simulink library "SimulinkLibrary"  (R2021b)
settings: Solver=VariableStepAuto  StartTime=0.0  StopTime=10.0  RelTol=1e-3
undefined symbols (not defined in the file): Ts, w0
libraries: canmsglib x6, $bdroot x5, sharedtransform x2, simulink x1
(part 2 of 3)

== system SimulinkLibrary/Sec ==
  SecContns : Inport
  Constant : Constant  Value=59  OutDataTypeStr=Inherit: Inherit via back propagation
  Constant1 : Constant  Value=0  OutDataTypeStr=Inherit: Inherit via back propagation
  Constant2 : Constant  Value=59  OutDataTypeStr=Inherit: Inherit via back propagation
  CountTo60 : Stateflow chart  TreatAsAtomicUnit=on
  Data Type Conversion1 : DataTypeConversion  OutDataTypeStr=boolean
  Equal : RelationalOperator  Operator===  OutDataTypeStr=boolean  RndMeth=Simplest
  Floor : Rounding
  Logical Operator : Logic  AllPortsSameDT=off  OutDataTypeStr=boolean
  Min : MinMax  Inputs=2
  Subtract : Sum  Inputs=+-
  Switch : Switch  Criteria=u2 ~= 0
  Unit Delay : UnitDelay  SampleTime=-1  HasFrameUpgradeWarning=on
  Unit Delay1 : UnitDelay  SampleTime=-1  HasFrameUpgradeWarning=on
  Sec : Outport
  wires:
  Constant1/1 -> Switch/1
  Constant/1 -> Min/2
  Floor/1 -> Unit Delay/1, Subtract/1  "floor"
  Logical Operator/1 -> Switch/2
  CountTo60/1(Out) -> Min/1  "Out"
  Min/1 -> Unit Delay1/1, Switch/3
  Constant2/1 -> Equal/2
  Unit Delay1/1 -> Equal/1
  Subtract/1 -> CountTo60/1(In), Data Type Conversion1/1  "In"
  Switch/1 -> Sec/1  "Seconds"
  Equal/1 -> Logical Operator/1
  SecContns/1 -> Floor/1  "SecContns"
  Unit Delay/1 -> Subtract/2
  Data Type Conversion1/1 -> Logical Operator/2

== system SimulinkLibrary/Vehicle Longitudinal model 1DOF ==
  FwF : Inport
  FwR : Inport  Port=2
  Grade : Inport  Port=3
  WindX : Inport  Port=4
  AirTempConstant : Constant  Value=T
  FExtConstant : Constant  Value=[0,0,0]
  MExtConstant : Constant  Value=[0,0,0]
  Subsystem : Subsystem
  Info : Outport  VectorParamsAs1DForOutWhenUnconnected=off
  xdot : Outport  Port=2  PortDimensions=1  VectorParamsAs1DForOutWhenUnconnected=off
  FzF : Outport  Port=3  PortDimensions=1  VectorParamsAs1DForOutWhenUnconnected=off
  FzR : Outport  Port=4  PortDimensions=1  VectorParamsAs1DForOutWhenUnconnected=off
  wires:
  Subsystem/4(FzR) -> FzR/1
  FwF/1 -> Subsystem/1(FwF)
  FwR/1 -> Subsystem/2(FwR)
  Subsystem/1(Info) -> Info/1
  AirTempConstant/1 -> Subsystem/7(Temp)
  WindX/1 -> Subsystem/4(wind)
  MExtConstant/1 -> Subsystem/6(MExt)
  Subsystem/3(FzF) -> FzF/1
  FExtConstant/1 -> Subsystem/5(FExt)
  Grade/1 -> Subsystem/3(Grade)
  Subsystem/2(xdot) -> xdot/1

== system SimulinkLibrary/Bundles/HwSelProc ==
  EX_DrvBtn_B_Psd : Inport
  EX_RvrsBtn_B_Psd : Inport  Port=2
  EX_NeutBtn_B_Psd : Inport  Port=3
  GearSelHeal_T_Pt : Inport  Port=4
  GearSelTrig_T_Pt : Inport  Port=5
  DMS_GearLock_B_Reqd : Inport  Port=6
  Chart : Stateflow chart  TreatAsAtomicUnit=on
  Chart1 : Stateflow chart  TreatAsAtomicUnit=on
  Chart2 : Stateflow chart  TreatAsAtomicUnit=on
  Chart3 : Stateflow chart  TreatAsAtomicUnit=on
      settings: PortSchema="{\"entries\":[{\"content\":{\"sides\":[{\"content\":{\"connectorIds\":[\"In2\",\"In1\",\"In3\",\"In4\"]},\"type\":\"ConnectorPlacement.EquallySpacedRectSide\",\"uuid\":\"b0ed4c9f-00b8-42d9-8b9d-c324759176df\"},{\"content\":{\"connectorIds\":[\"Out1\"],\"side\":\"RIGHT\"},\"type\":\"ConnectorPlacement.EquallySpacedRectSide\",\"uuid\":\"c1b9fe74-1ccd-4df0-a60b-616e1fa68e70\"},{\"content\":{\"connectorIds\":[],\"side\":\"TOP\"},\"type\":\"ConnectorPlacement.EquallySpacedRectSide\",\"uuid\":\"07870c33-9b1f-4d61-9115-d019d8c5b702\"}]},\"type\":\"ConnectorPlacement.EquallySpacedConnector\",\"uuid\":\"fdc9da14-557c-4fc0-875a-2215d5d98432\"}],\"packageUris\":[\"http://schema.mathworks.com/mf0/Connector/R2020b\"],\"version\":\"1.0\"}"
  DMS_HwEltGearPosn_Zs : Outport
  wires:
  Chart3/1(DMS_HwEltGearPosn_Zs) -> DMS_HwEltGearPosn_Zs/1
  DMS_GearLock_B_Reqd/1 -> Chart3/4(DMS_GearLock_B_Reqd)  "DMS_GearLock_B_Reqd"
  Chart2/1(Out) -> Chart3/3(NeutBtn_B_PsdFild)  "NeutBtn_B_PsdFild"
  Chart1/1(Out) -> Chart3/1(DrvBtn_B_PsdFild)  "DrvBtn_B_PsdFild"
  Chart/1(Out) -> Chart3/2(RvrsBtn_B_PsdFild)  "DrvBtn_B_PsdFild"
  [GearSelTrig_T_Pt] -> Chart2/3(TriggerTime)
  [GearSelHeal_T_Pt] -> Chart2/2(HealTime)
  [GearSelTrig_T_Pt] -> Chart1/3(TriggerTime)
  [GearSelHeal_T_Pt] -> Chart1/2(HealTime)
  [GearSelTrig_T_Pt] -> Chart/3(TriggerTime)
  [GearSelHeal_T_Pt] -> Chart/2(HealTime)
  EX_NeutBtn_B_Psd/1 -> Chart2/1(In)  "EX_NeutBtn_B_Psd"
  EX_RvrsBtn_B_Psd/1 -> Chart1/1(In)  "EX_RvrsBtn_B_Psd"
  EX_DrvBtn_B_Psd/1 -> Chart/1(In)  "EX_DrvBtn_B_Psd"
  GearSelHeal_T_Pt/1 -> [GearSelHeal_T_Pt]  "GearSelHeal_T_Pt"
  GearSelTrig_T_Pt/1 -> [GearSelTrig_T_Pt]  "GearSelTrig_T_Pt"

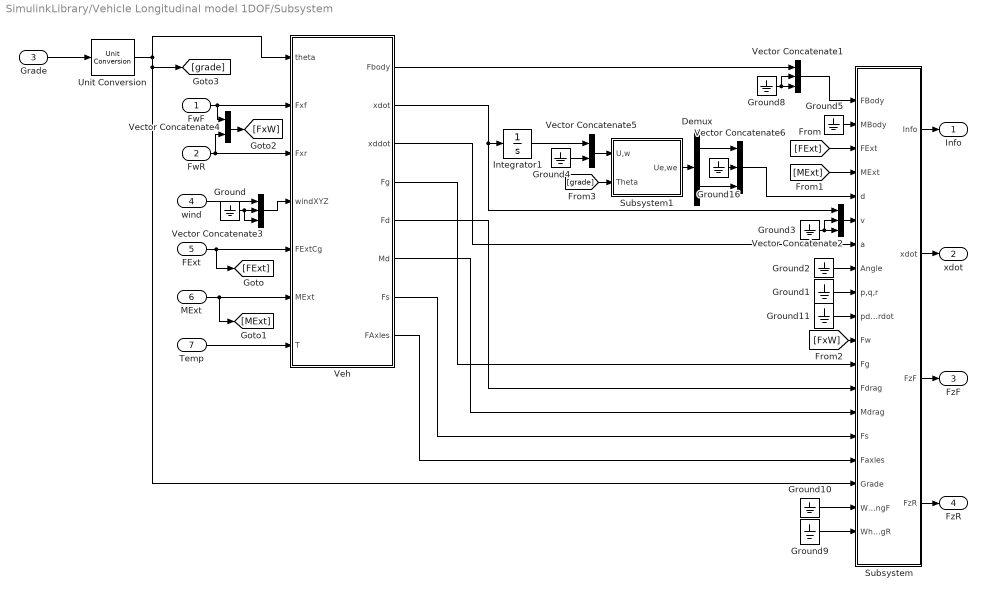
== system SimulinkLibrary/Vehicle Longitudinal model 1DOF/Subsystem ==
  FwF : Inport  Unit=N
  FwR : Inport  Port=2  Unit=N
  Grade : Inport  Port=3  Unit=deg
  wind : Inport  Port=4  Unit=m/s
  FExt : Inport  Port=5  Unit=N
  MExt : Inport  Port=6  Unit=N*m
  Temp : Inport  Port=7  OutMin=eps  Unit=K
  Demux : Demux  Outputs=2
  Ground{,1..5,8..11,16} (11 alike) : Ground
  Integrator1 : Integrator  InitialCondition=x_o
  Subsystem : Subsystem
  Subsystem1 : Subsystem
  Unit Conversion : UnitConversion
  Vector Concatenate{1..3,6} (4 alike) : Concatenate  NumInputs=3
  Vector Concatenate4 : Concatenate
  Vector Concatenate5 : Concatenate
  Veh : Subsystem
  Info : Outport  VectorParamsAs1DForOutWhenUnconnected=off
  xdot : Outport  Port=2  Unit=m/s  VectorParamsAs1DForOutWhenUnconnected=off
  FzF : Outport  Port=3  Unit=N  VectorParamsAs1DForOutWhenUnconnected=off
  FzR : Outport  Port=4  Unit=N  VectorParamsAs1DForOutWhenUnconnected=off
  wires:
  MExt/1 -> Veh/6(MExt), [MExt]
  [MExt] -> Subsystem/4(MExt)
  Veh/7(Fs) -> Subsystem/15(Fs)
  Ground9/1 -> Subsystem/19(WhlAngR)
  Vector Concatenate5/1 -> Subsystem1/1(U,w)
  Ground4/1 -> Vector Concatenate5/2
  Ground16/1 -> Vector Concatenate6/2
  Veh/4(Fg) -> Subsystem/12(Fg)
  Demux/1 -> Vector Concatenate6/1
  Subsystem1/1(Ue,we) -> Demux/1
  Vector Concatenate3/1 -> Veh/4(windXYZ)
  Veh/5(Fd) -> Subsystem/13(Fdrag)
  Unit Conversion/1 -> Veh/1(theta), Subsystem/17(Grade), [grade]
  Ground5/1 -> Subsystem/2(MBody)
  [FxW] -> Subsystem/11(Fw)
  Ground11/1 -> Subsystem/10(pdot,qdot,rdot)
  Vector Concatenate2/1 -> Subsystem/6(v)
  Veh/3(xddot) -> Subsystem/7(a)
  Veh/6(Md) -> Subsystem/14(Mdrag)
  Demux/2 -> Vector Concatenate6/3
  FwF/1 -> Veh/2(Fxf), Vector Concatenate4/1
  Ground1/1 -> Subsystem/9(p,q,r)
  Subsystem/1(Info) -> Info/1
  Ground10/1 -> Subsystem/18(WhlAngF)
  FwR/1 -> Veh/3(Fxr), Vector Concatenate4/2
  Subsystem/4(FzR) -> FzR/1
  Vector Concatenate4/1 -> [FxW]
  Veh/8(FAxles) -> Subsystem/16(Faxles)
  Veh/2(xdot) -> Integrator1/1, Vector Concatenate2/1
  Ground3/1 -> Vector Concatenate2/3, Vector Concatenate2/2
  Grade/1 -> Unit Conversion/1
  Subsystem/2(xdot) -> xdot/1
  Subsystem/3(FzF) -> FzF/1
  Ground2/1 -> Subsystem/8(Angle)
  Integrator1/1 -> Vector Concatenate5/1
  [FExt] -> Subsystem/3(FExt)
  Vector Concatenate1/1 -> Subsystem/1(FBody)
  FExt/1 -> Veh/5(FExtCg), [FExt]
  Veh/1(Fbody) -> Vector Concatenate1/1
  Temp/1 -> Veh/7(T)
  Vector Concatenate6/1 -> Subsystem/5(d)
  [grade] -> Subsystem1/2(Theta)
  Ground8/1 -> Vector Concatenate1/2, Vector Concatenate1/3
  wind/1 -> Vector Concatenate3/1
  Ground/1 -> Vector Concatenate3/3, Vector Concatenate3/2

== system SimulinkLibrary/Vehicle Longitudinal model 1DOF/Subsystem/Subsystem ==
  FBody : Inport
  MBody : Inport  Port=2  Unit=N*m
  FExt : Inport  Port=3  Unit=N
  MExt : Inport  Port=4  Unit=N*m
  d : Inport  Port=5  Unit=m
  v : Inport  Port=6  Unit=m/s
  a : Inport  Port=7  Unit=m/s^2
  Angle : Inport  Port=8  Unit=rad
  p,q,r : Inport  Port=9  Unit=rad/s
  pdot,qdot,rdot : Inport  Port=10  Unit=rad/s^2
  Fw : Inport  Port=11
  Fg : Inport  Port=12  Unit=N
  Fdrag : Inport  Port=13  Unit=N
  Mdrag : Inport  Port=14  Unit=N*m
  Fs : Inport  Port=15  Unit=N
  Faxles : Inport  Port=16  Unit=N
  Grade : Inport  Port=17  Unit=rad
  WhlAngF : Inport  Port=18  Unit=rad
  WhlAngR : Inport  Port=19  Unit=rad
  Bus Creator16 : BusCreator  Inputs=3
  Bus Selector : BusSelector  OutputSignals=BdyFrm.Cg.Vel.xdot
  Bus Selector1 : BusSelector  OutputSignals=InertFrm
  Bus Selector2 : BusSelector  OutputSignals=BdyFrm
  Selector : Selector  InputPortWidth=3  IndexOptions=Index vector (dialog)  Indices=[1 3]  OutputSizes=1
  Selector1 : Selector  InputPortWidth=3  IndexOptions=Index vector (dialog)  Indices=[2]  OutputSizes=1
  Selector2 : Selector  InputPortWidth=3  IndexOptions=Index vector (dialog)  Indices=[1 3]  OutputSizes=1
  Subsystem : Subsystem
  Subsystem1 : Subsystem
  Subsystem2 : Subsystem
  Subsystem3 : Subsystem
  Subsystem4 : Subsystem
  Subsystem5 : Subsystem
  Info : Outport  VectorParamsAs1DForOutWhenUnconnected=off
  xdot : Outport  Port=2  VectorParamsAs1DForOutWhenUnconnected=off
  FzF : Outport  Port=3  VectorParamsAs1DForOutWhenUnconnected=off
  FzR : Outport  Port=4  VectorParamsAs1DForOutWhenUnconnected=off
  wires:
  Bus Selector/1 -> xdot/1  "<xdot>"
  Fg/1 -> Subsystem1/4(Fg)
  Subsystem/1(Cg) -> Subsystem5/2(BdyFrmCg)  "Cg"
  Grade/1 -> Subsystem3/4(Grade)
  Subsystem2/1(Moments) -> Subsystem5/5(Moments), Subsystem4/4(Moments)  "Moments"
  Subsystem1/3(FzR) -> FzR/1
  Bus Creator16/1 -> [InfoBus], Bus Selector/1, Info/1  "Info"
  MBody/1 -> Subsystem2/1(MBody)
  Selector1/1 -> Subsystem3/3(theta)
  Fw/1 -> Subsystem1/1(Fw), Subsystem4/6(Fw)
  Subsystem1/1(Forces) -> Subsystem5/3(Forces), Subsystem4/3(Forces)  "Forces"
  a/1 -> Subsystem/3(a)
  Fs/1 -> Subsystem4/5(Fsusp)
  MExt/1 -> Subsystem2/3(MExt)
  Mdrag/1 -> Subsystem2/2(Mdrag)
  Selector/1 -> Subsystem3/2(U,w)
  Bus Selector2/1 -> Subsystem4/2(BodyCg)  "<BdyFrm>"
  Selector2/1 -> Subsystem3/1(X,Z)
  Subsystem4/1(Pwr) -> Subsystem5/4(Power)  "Pwr"
  Subsystem5/1(InertFrm) -> Bus Creator16/1  "InertFrm"
  WhlAngR/1 -> Subsystem5/7(WhlAngR)
  d/1 -> Selector2/1
  Angle/1 -> Selector1/1
  Bus Selector1/1 -> Subsystem4/1(InertCg)  "<InertFrm>"
  pdot,qdot,rdot/1 -> Subsystem/4(pdot,qdot,rdot)
  [InfoBus] -> Bus Selector2/1, Bus Selector1/1
  p,q,r/1 -> Subsystem/2(p,q,r)
  Subsystem5/3(PwrInfo) -> Bus Creator16/3  "PwrInfo"
  v/1 -> Subsystem/1(v), Selector/1
  WhlAngF/1 -> Subsystem5/6(WhlAngF)
  FBody/1 -> Subsystem1/2(FBody)
  Fdrag/1 -> Subsystem1/3(Fdrag)
  Subsystem3/1(Cg) -> Subsystem5/1(InertCg)  "Cg"
  Faxles/1 -> Subsystem1/5(Faxles)
  FExt/1 -> Subsystem1/6(FExt)
  Subsystem5/2(BdyFrm) -> Bus Creator16/2  "BdyFrm"
  Subsystem1/2(FzF) -> FzF/1

== system SimulinkLibrary/Vehicle Longitudinal model 1DOF/Subsystem/Subsystem1 ==
  U,w : Inport
  Theta : Inport  Port=2
  Constant : Constant  Value=0
  Mux3 : Mux  Inputs=3
  Mux4 : Mux  Inputs=3
  Product : Product  Multiplication=Matrix(*)  SaturateOnIntegerOverflow=on  OutDataTypeStr=Inherit: Same as first input
  Rotation Angles to Direction Cosine Matrix : sharedtransform/Rotation Angles to Direction Cosine Matrix  rotationOrder=ZYX  aMode=aMode
      settings: SourceProductBaseCode=AE,PW,DR,MT,UV,VE
  Selector : Selector  InputPortWidth=2  IndexOptions=Index vector (dialog)  Indices=1  OutputSizes=1
  Selector1 : Selector  InputPortWidth=3  IndexOptions=Index vector (dialog)  Indices=[1 3]  OutputSizes=1
  Selector2 : Selector  InputPortWidth=2  IndexOptions=Index vector (dialog)  Indices=2  OutputSizes=1
  Transpose : Math  Operator=transpose  SignedPower=on  SaturateOnIntegerOverflow=on
  Ue,we : Outport  Unit=m/s  VectorParamsAs1DForOutWhenUnconnected=off
  wires:
  U,w/1 -> Selector/1, Selector2/1
  Selector2/1 -> Mux4/3
  Rotation Angles to Direction Cosine Matrix/1 -> Transpose/1
  Constant/1 -> Mux3/1, Mux4/2, Mux3/3
  Mux3/1 -> Rotation Angles to Direction Cosine Matrix/1
  Selector1/1 -> Ue,we/1
  Product/1 -> Selector1/1
  Selector/1 -> Mux4/1
  Theta/1 -> Mux3/2
  Transpose/1 -> Product/1
  Mux4/1 -> Product/2

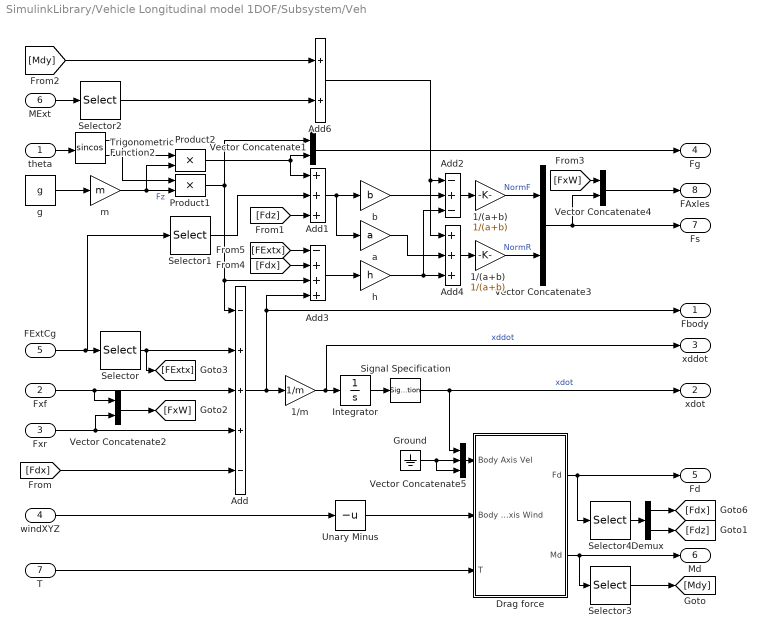
== system SimulinkLibrary/Vehicle Longitudinal model 1DOF/Subsystem/Veh ==
  theta : Inport  Unit=rad
  Fxf : Inport  Port=2
  Fxr : Inport  Port=3
  windXYZ : Inport  Port=4
  FExtCg : Inport  Port=5
  MExt : Inport  Port=6
  T : Inport  Port=7
  1/(a+b) : Gain  Gain=1/(a+b)
  "1/(a+b) " : Gain  Gain=1/(a+b)
  1/m : Gain  Gain=1/m
  Add : Sum  Inputs=-+++-
  Add1 : Sum  Inputs=+++
  Add2 : Sum  Inputs=-+-
  Add3 : Sum  Inputs=-+++
  Add4 : Sum  Inputs=+++
  Add6 : Sum
  Demux : Demux  Outputs=2
  Drag force : Subsystem  mask{A=Af, beta_w=[-1,1], Cd=Cd, Cs=[0,0], Cl=Cl, Cpm=Cpm, Lcpm=a+b, Crm=[0,0], Cym=[0,0], R=287.058, Pabs=Pabs}
      mask prompts: A "Effective area, A [m^s2]:"; beta_w "Relative wind angle vector, beta_w [rad]:"; Cd "Longitudinal drag coefficient, Cd [-]:"; Cs "Side force coefficient data, Cs [-]:"; Cl "Lift coefficient, Cl [-]:"; Cpm "Pitch moment coefficient, Cpm [-]:"; Lcpm "Pitch moment length, Lcpm"; Crm "Roll moment coefficient data, Crm [-]:"; Cym "Yaw moment coefficient data, Cym [-]:"; R "Gas constant, R [J/(kg*K)]:"; Pabs "Absoulte pressure, Pabs [Pa]:"
  Ground : Ground
  Integrator : Integrator  InitialCondition=xdot_o
  Product1 : Product
  Product2 : Product
  Selector : Selector  InputPortWidth=3  IndexOptions=Index vector (dialog)  Indices=[1]  OutputSizes=1
  Selector1 : Selector  InputPortWidth=3  IndexOptions=Index vector (dialog)  Indices=[3]  OutputSizes=1
  Selector2 : Selector  InputPortWidth=3  IndexOptions=Index vector (dialog)  Indices=[2]  OutputSizes=1
  Selector3 : Selector  InputPortWidth=3  IndexOptions=Index vector (dialog)  Indices=[2]  OutputSizes=1
  Selector4 : Selector  InputPortWidth=3  IndexOptions=Index vector (dialog)  Indices=[1 3]  OutputSizes=1
  Signal Specification : SignalSpecification  Unit=m/s  Dimensions=1
  Trigonometric Function2 : Trigonometry  Operator=sincos
  Unary Minus : UnaryMinus
  Vector Concatenate1 : Concatenate
  Vector Concatenate2 : Concatenate
  Vector Concatenate3 : Concatenate
  Vector Concatenate4 : Concatenate  Mode=Multidimensional array  ConcatenateDimension=2
  Vector Concatenate5 : Concatenate  NumInputs=3
  a : Gain  Gain=a
  b : Gain  Gain=b
  g : Constant  Value=g
  h : Gain  Gain=h
  m : Gain  Gain=m
  Fbody : Outport  VectorParamsAs1DForOutWhenUnconnected=off
  xdot : Outport  Port=2  VectorParamsAs1DForOutWhenUnconnected=off
  xddot : Outport  Port=3  VectorParamsAs1DForOutWhenUnconnected=off
  Fg : Outport  Port=4  VectorParamsAs1DForOutWhenUnconnected=off
  Fd : Outport  Port=5  VectorParamsAs1DForOutWhenUnconnected=off
  Md : Outport  Port=6  VectorParamsAs1DForOutWhenUnconnected=off
  Fs : Outport  Port=7  VectorParamsAs1DForOutWhenUnconnected=off
  FAxles : Outport  Port=8  VectorParamsAs1DForOutWhenUnconnected=off
  wires:
  FExtCg/1 -> Selector/1, Selector1/1
  1/(a+b)/1 -> Vector Concatenate3/1  "NormF"
  Fxf/1 -> Vector Concatenate2/1, Add/3
  Add/1 -> 1/m/1, Fbody/1, Add3/4
  Unary Minus/1 -> Drag force/2(Body Axis Wind)
  Vector Concatenate2/1 -> [FxW]
  Ground/1 -> Vector Concatenate5/2, Vector Concatenate5/3
  Product2/1 -> Add1/1, Vector Concatenate1/2
  Selector/1 -> Add/2, [FExtx]
  Trigonometric Function2/2 -> Product2/1
  Add2/1 -> 1/(a+b)/1
  Vector Concatenate5/1 -> Drag force/1(Body Axis Vel)
  Vector Concatenate1/1 -> Fg/1
  Selector4/1 -> Demux/1
  b/1 -> Add2/2
  1/m/1 -> Integrator/1, xddot/1  "xddot"
  Add1/1 -> b/1, a/1
  Integrator/1 -> Signal Specification/1
  Demux/2 -> [Fdz]
  Vector Concatenate3/1 -> Fs/1, Vector Concatenate4/2
  T/1 -> Drag force/3(T)
  theta/1 -> Trigonometric Function2/1
  [Fdx] -> Add3/2
  Selector2/1 -> Add6/2
  m/1 -> Product1/2, Product2/2  "Fz"
  Selector1/1 -> Add1/2
  h/1 -> Add4/3, Add2/3
  MExt/1 -> Selector2/1
  [FxW] -> Vector Concatenate4/1
  Add4/1 -> "1/(a+b) "/1
  Vector Concatenate4/1 -> FAxles/1
  [Fdx] -> Add/5
  Add6/1 -> Add2/1, Add4/1
  Drag force/1(Fd) -> Fd/1, Selector4/1
  Drag force/2(Md) -> Md/1, Selector3/1
  Trigonometric Function2/1 -> Product1/1
  "1/(a+b) "/1 -> Vector Concatenate3/2  "NormR"
  Fxr/1 -> Vector Concatenate2/2, Add/4
  Selector3/1 -> [Mdy]
  Demux/1 -> [Fdx]
  [Fdz] -> Add1/3
  windXYZ/1 -> Unary Minus/1
  [Mdy] -> Add6/1
  Product1/1 -> Add3/3, Add/1, Vector Concatenate1/1
  a/1 -> Add4/2
  Add3/1 -> h/1
  Signal Specification/1 -> Vector Concatenate5/1, xdot/1  "xdot"
  g/1 -> m/1
  [FExtx] -> Add3/1

== system SimulinkLibrary/Vehicle Longitudinal model 1DOF/Subsystem/Subsystem/Subsystem ==
  v : Inport  Unit=m/s
  p,q,r : Inport  Port=2  Unit=rad/s
  a : Inport  Port=3  Unit=m/s^2
  pdot,qdot,rdot : Inport  Port=4
  Subsystem : Subsystem
  Cg : Outport  VectorParamsAs1DForOutWhenUnconnected=off
  wires:
  Subsystem/1(Cg) -> Cg/1
  v/1 -> Subsystem/1(v)
  p,q,r/1 -> Subsystem/2(p,q,r)
  a/1 -> Subsystem/3(a)
  pdot,qdot,rdot/1 -> Subsystem/4(pdot,qdot,rdot)

== system SimulinkLibrary/Vehicle Longitudinal model 1DOF/Subsystem/Subsystem/Subsystem1 ==
  Fw : Inport
  FBody : Inport  Port=2
  Fdrag : Inport  Port=3
  Fg : Inport  Port=4
  Faxles : Inport  Port=5
  FExt : Inport  Port=6
  Subsystem : Subsystem
  Terminator : Terminator
  Forces : Outport  VectorParamsAs1DForOutWhenUnconnected=off
  FzF : Outport  Port=2  VectorParamsAs1DForOutWhenUnconnected=off
  FzR : Outport  Port=3  VectorParamsAs1DForOutWhenUnconnected=off
  wires:
  Fdrag/1 -> Subsystem/1(Fdrag)
  FBody/1 -> Subsystem/5(FBody)
  Fg/1 -> Subsystem/2(Fg)
  Faxles/1 -> Subsystem/3(Faxles)
  FExt/1 -> Subsystem/4(FExt)
  Subsystem/3(FzR) -> FzR/1
  Subsystem/2(FzF) -> FzF/1
  Subsystem/1(Forces) -> Forces/1
  Fw/1 -> Terminator/1

== system SimulinkLibrary/Vehicle Longitudinal model 1DOF/Subsystem/Subsystem/Subsystem2 ==
  MBody : Inport
  Mdrag : Inport  Port=2  PortDimensions=3
  MExt : Inport  Port=3  PortDimensions=3
  Bus Creator{1,3,7,24} (4 alike) : BusCreator  Inputs=3
  Demux : Demux  Outputs=3
  Demux1 : Demux  Outputs=3
  Demux2 : Demux  Outputs=3
  Signal Specification{1..8,23} (9 alike) : SignalSpecification  Unit=N*m
  Moments : Outport  VectorParamsAs1DForOutWhenUnconnected=off
  wires:
  Signal Specification2/1 -> Bus Creator24/3  "Mz"
  Signal Specification8/1 -> Bus Creator3/1  "Mx"
  Signal Specification6/1 -> Bus Creator3/2  "My"
  Signal Specification4/1 -> Bus Creator1/3  "Mz"
  Bus Creator1/1 -> Bus Creator7/2  "Drag"
  Signal Specification5/1 -> Bus Creator1/1  "Mx"
  Demux1/1 -> Signal Specification5/1
  Demux1/3 -> Signal Specification4/1
  Signal Specification7/1 -> Bus Creator3/3  "Mz"
  Bus Creator7/1 -> Moments/1  "Moments"
  Signal Specification3/1 -> Bus Creator1/2  "My"
  MBody/1 -> Demux/1
  Demux1/2 -> Signal Specification3/1
  Mdrag/1 -> Demux1/1
  Demux/3 -> Signal Specification2/1
  MExt/1 -> Demux2/1
  Demux/1 -> Signal Specification23/1
  Signal Specification23/1 -> Bus Creator24/1  "Mx"
  Signal Specification1/1 -> Bus Creator24/2  "My"
  Demux2/3 -> Signal Specification7/1
  Bus Creator3/1 -> Bus Creator7/3  "Ext"
  Demux/2 -> Signal Specification1/1
  Demux2/1 -> Signal Specification8/1
  Bus Creator24/1 -> Bus Creator7/1  "Body"
  Demux2/2 -> Signal Specification6/1

== system SimulinkLibrary/Vehicle Longitudinal model 1DOF/Subsystem/Subsystem/Subsystem3 ==
  X,Z : Inport  Unit=m
  U,w : Inport  Port=2
  theta : Inport  Port=3
  Grade : Inport  Port=4
  Add : Sum
  Bus Creator{6..7,11,24} (4 alike) : BusCreator  Inputs=3
  Constant{1..2,10,12} (4 alike) : Constant  Value=0
  Demux : Demux  Outputs=2
  Demux5 : Demux  Outputs=2
  Signal Specification1 : SignalSpecification  Unit=rad
  Signal Specification2 : SignalSpecification  Unit=rad
  Signal Specification23 : SignalSpecification  Unit=m
  Signal Specification24 : SignalSpecification  Unit=m
  Signal Specification25 : SignalSpecification  Unit=m
  Signal Specification26 : SignalSpecification  Unit=rad
  Signal Specification7 : SignalSpecification  Unit=m/s
  Signal Specification8 : SignalSpecification  Unit=m/s
  Signal Specification9 : SignalSpecification  Unit=m/s
  Subsystem : Subsystem
  Cg : Outport  VectorParamsAs1DForOutWhenUnconnected=off
  wires:
  X,Z/1 -> Demux5/1  "XZ"
  Signal Specification1/1 -> Bus Creator11/1  "phi"
  Grade/1 -> Add/1
  Signal Specification26/1 -> Bus Creator11/2  "theta"
  theta/1 -> Signal Specification26/1, Add/2
  Constant1/1 -> Signal Specification1/1
  Constant12/1 -> Signal Specification24/1  "Y"
  Constant2/1 -> Signal Specification2/1
  U,w/1 -> Subsystem/1(U,w)
  Demux/2 -> Signal Specification9/1  "Zdot"
  Bus Creator7/1 -> Cg/1  "Cg"
  Add/1 -> Subsystem/2(Theta)
  Bus Creator11/1 -> Bus Creator7/3  "Ang"
  Subsystem/1(Ue,we) -> Demux/1
  Signal Specification7/1 -> Bus Creator6/2  "Ydot"
  Constant10/1 -> Signal Specification7/1
  Signal Specification23/1 -> Bus Creator24/1  "X"
  Bus Creator24/1 -> Bus Creator7/1  "Disp"
  Signal Specification8/1 -> Bus Creator6/1  "Xdot"
  Demux/1 -> Signal Specification8/1  "Xdot"
  Signal Specification25/1 -> Bus Creator24/3  "Z"
  Bus Creator6/1 -> Bus Creator7/2  "Vel"
  Signal Specification9/1 -> Bus Creator6/3  "Zdot"
  Demux5/1 -> Signal Specification23/1  "X"
  Demux5/2 -> Signal Specification25/1  "Z"
  Signal Specification24/1 -> Bus Creator24/2  "Y"
  Signal Specification2/1 -> Bus Creator11/3  "psi"

== system SimulinkLibrary/Vehicle Longitudinal model 1DOF/Subsystem/Subsystem/Subsystem4 ==
  InertCg : Inport
  BodyCg : Inport  Port=2
  Forces : Inport  Port=3
  Moments : Inport  Port=4
  Fsusp : Inport  Port=5
  Fw : Inport  Port=6
  Subsystem : Subsystem
  Terminator : Terminator
  Terminator1 : Terminator
  Pwr : Outport  VectorParamsAs1DForOutWhenUnconnected=off
  wires:
  Fw/1 -> Terminator1/1
  Fsusp/1 -> Terminator/1
  InertCg/1 -> Subsystem/1(InertCg)
  BodyCg/1 -> Subsystem/2(BodyCg)
  Forces/1 -> Subsystem/3(Forces)
  Moments/1 -> Subsystem/4(Moments)
  Subsystem/1(Pwr) -> Pwr/1

== system SimulinkLibrary/Vehicle Longitudinal model 1DOF/Subsystem/Subsystem/Subsystem5 ==
  InertCg : Inport
  BdyFrmCg : Inport  Port=2
  Forces : Inport  Port=3
  Power : Inport  Port=4
  Moments : Inport  Port=5
  WhlAngF : Inport  Port=6
  WhlAngR : Inport  Port=7
  Subsystem : Subsystem
  InertFrm : Outport  VectorParamsAs1DForOutWhenUnconnected=off
  BdyFrm : Outport  Port=2  VectorParamsAs1DForOutWhenUnconnected=off
  PwrInfo : Outport  Port=3  VectorParamsAs1DForOutWhenUnconnected=off
  wires:
  InertCg/1 -> Subsystem/1(InertCg)
  Subsystem/1(InertFrm) -> InertFrm/1
  Subsystem/2(BdyFrm) -> BdyFrm/1
  Subsystem/3(PwrInfo) -> PwrInfo/1
  BdyFrmCg/1 -> Subsystem/2(BdyFrmCg)
  Forces/1 -> Subsystem/3(Forces)
  Power/1 -> Subsystem/4(Power)
  Moments/1 -> Subsystem/5(Moments)
  WhlAngF/1 -> Subsystem/6(WhlAngF)
  WhlAngR/1 -> Subsystem/7(WhlAngR)

== system SimulinkLibrary/Vehicle Longitudinal model 1DOF/Subsystem/Veh/Drag force ==
  Body Axis Vel : Inport
  Body Axis Wind : Inport  Port=2
  T : Inport  Port=3  OutMin=1
  .5.*A.*Pabs./R./T : Gain  Gain=.5.*A.*Pabs./R
  Add1 : Sum  Inputs=+-
  Constant : Constant  Value=Cd
  Constant1 : Constant  Value=Cl
  Constant2 : Constant  Value=Cpm
  Constant3 : Constant  Value=Lcpm
  Constant4 : Constant  Value=ones(1,3)
  Crm : Lookup_n-D  NumberOfTableDimensions=1  BreakpointsForDimension1=[-1 1]  Table=[0 0]  InternalRulePriority=Speed  RndMeth=Simplest  InputSameDT=on
  Cs : Lookup_n-D  NumberOfTableDimensions=1  BreakpointsForDimension1=beta_w  Table=Cs  ExtrapMethod=Clip  InternalRulePriority=Speed  RndMeth=Simplest  InputSameDT=on
  Cym : Lookup_n-D  NumberOfTableDimensions=1  BreakpointsForDimension1=beta_w  Table=Cym  InternalRulePriority=Speed  RndMeth=Simplest  InputSameDT=on
  Demux : Demux  Outputs=2
  Product{,2..5} (5 alike) : Product
  Product1 : Product  Inputs=**/
  Selector : Selector  InputPortWidth=3  IndexOptions=Index vector (dialog)  Indices=[2 1]  OutputSizes=1
  Selector1 : Selector  InputPortWidth=3  IndexOptions=Index vector (dialog)  Indices=[1]  OutputSizes=1
  Selector2 : Selector  InputPortWidth=6  IndexOptions=Index vector (dialog)  Indices=[4:6]  OutputSizes=1
  Selector3 : Selector  InputPortWidth=6  IndexOptions=Index vector (dialog)  Indices=[1:3]  OutputSizes=1
  Sqrt : Sqrt  SaturateOnIntegerOverflow=on
  Sum of Elements : Sum  Inputs=+
  Switch : Switch  ZeroCross=off
  Trigonometric Function : Trigonometry  Operator=atan2  OutputSignalType=real
  Unary Minus : UnaryMinus
  Vector Concatenate : Concatenate  NumInputs=6
  Fd : Outport  VectorParamsAs1DForOutWhenUnconnected=off
  Md : Outport  Port=2  VectorParamsAs1DForOutWhenUnconnected=off
  wires:
  Selector1/1 -> Product5/1
  T/1 -> Product1/3
  Demux/1 -> Trigonometric Function/1
  Constant4/1 -> Unary Minus/1, Switch/1
  Constant2/1 -> Product5/2
  Vector Concatenate/1 -> Product1/2
  [windDir] -> Selector1/1
  Switch/1 -> [windDir], Product3/1
  Constant3/1 -> Product4/2
  Crm/1 -> Vector Concatenate/4
  Unary Minus/1 -> Switch/3
  Body Axis Wind/1 -> Add1/2
  Selector3/1 -> Product3/2
  Cym/1 -> Vector Concatenate/6
  Selector2/1 -> Product4/1
  Product5/1 -> Vector Concatenate/5
  Constant1/1 -> Vector Concatenate/3
  Product4/1 -> Md/1
  Product/1 -> Sum of Elements/1
  Product2/1 -> Product1/1
  Selector/1 -> Demux/1
  Product1/1 -> .5.*A.*Pabs./R./T/1
  Trigonometric Function/1 -> Cs/1, Crm/1, Cym/1
  Body Axis Vel/1 -> Add1/1
  Add1/1 -> Switch/2, Selector/1, Product/2, Product/1
  Demux/2 -> Trigonometric Function/2
  Product3/1 -> Fd/1
  Constant/1 -> Vector Concatenate/1
  Cs/1 -> Vector Concatenate/2
  .5.*A.*Pabs./R./T/1 -> Selector3/1, Selector2/1
  Sqrt/1 -> Product2/1, Product2/2
  Sum of Elements/1 -> Sqrt/1

== system SimulinkLibrary/Vehicle Longitudinal model 1DOF/Subsystem/Subsystem/Subsystem/Subsystem ==
  v : Inport
  p,q,r : Inport  Port=2
  a : Inport  Port=3
  pdot,qdot,rdot : Inport  Port=4
  Bus Creator{1..2,13..14,21} (5 alike) : BusCreator  Inputs=3
  Bus Creator15 : BusCreator  Inputs=5
  Constant1 : Constant  Value=0
  Constant11 : Constant  Value=0
  Constant8 : Constant  Value=0
  Demux1 : Demux  Outputs=3
  Demux2 : Demux  Outputs=3
  Demux3 : Demux  Outputs=3
  Integrator3 : Integrator  InitialCondition=xdot_o
  Signal Specification1 : SignalSpecification  Unit=rad/s^2
  Signal Specification10 : SignalSpecification  Unit=m
  Signal Specification11 : SignalSpecification  Unit=m/s
  Signal Specification12 : SignalSpecification  Unit=m
  Signal Specification13 : SignalSpecification  Unit=m
  Signal Specification2 : SignalSpecification  Unit=gn
  Signal Specification27 : SignalSpecification  Unit=rad/s
  Signal Specification28 : SignalSpecification  Unit=rad/s
  Signal Specification29 : SignalSpecification  Unit=rad/s
  Signal Specification3 : SignalSpecification  Unit=gn
  Signal Specification4 : SignalSpecification  Unit=gn
  Signal Specification5 : SignalSpecification  Unit=m/s
  Signal Specification6 : SignalSpecification  Unit=m/s
  Signal Specification7 : SignalSpecification  Unit=rad/s^2
  Signal Specification8 : SignalSpecification  Unit=rad/s^2
  Unit Conversion : UnitConversion
  Cg : Outport  VectorParamsAs1DForOutWhenUnconnected=off
  wires:
  a/1 -> Unit Conversion/1
  Signal Specification3/1 -> Bus Creator2/1  "ax"
  Bus Creator21/1 -> Bus Creator15/1  "Disp"
  Bus Creator14/1 -> Bus Creator15/2  "Vel"
  Demux2/2 -> Signal Specification5/1
  v/1 -> Demux2/1
  Signal Specification12/1 -> Bus Creator21/2  "y"
  Signal Specification5/1 -> Bus Creator14/2  "ydot"
  Demux2/3 -> Signal Specification6/1
  Signal Specification6/1 -> Bus Creator14/3  "zdot"
  Demux3/3 -> Signal Specification29/1
  Signal Specification11/1 -> Bus Creator14/1  "xdot"
  Signal Specification2/1 -> Bus Creator2/2  "ay"
  Signal Specification29/1 -> Bus Creator13/3  "r"
  pdot,qdot,rdot/1 -> Demux1/1
  Bus Creator15/1 -> Cg/1  "Cg"
  Signal Specification13/1 -> Bus Creator21/3  "z"
  Signal Specification28/1 -> Bus Creator13/1  "p"
  Demux2/1 -> Integrator3/1, Signal Specification11/1
  Bus Creator13/1 -> Bus Creator15/3  "AngVel"
  Signal Specification4/1 -> Bus Creator2/3  "az"
  Constant8/1 -> Signal Specification2/1
  Constant1/1 -> Signal Specification4/1
  Constant11/1 -> Signal Specification13/1, Signal Specification12/1
  Signal Specification10/1 -> Bus Creator21/1  "x"
  Signal Specification1/1 -> Bus Creator1/2  "qdot"
  Demux3/2 -> Signal Specification27/1
  Demux1/2 -> Signal Specification1/1
  Integrator3/1 -> Signal Specification10/1  "x"
  Signal Specification7/1 -> Bus Creator1/1  "pdot"
  Demux3/1 -> Signal Specification28/1
  Demux1/1 -> Signal Specification7/1
  Bus Creator2/1 -> Bus Creator15/4  "Acc"
  Signal Specification8/1 -> Bus Creator1/3  "rdot"
  Demux1/3 -> Signal Specification8/1
  Signal Specification27/1 -> Bus Creator13/2  "q"
  p,q,r/1 -> Demux3/1
  Bus Creator1/1 -> Bus Creator15/5  "AngAcc"
  Unit Conversion/1 -> Signal Specification3/1

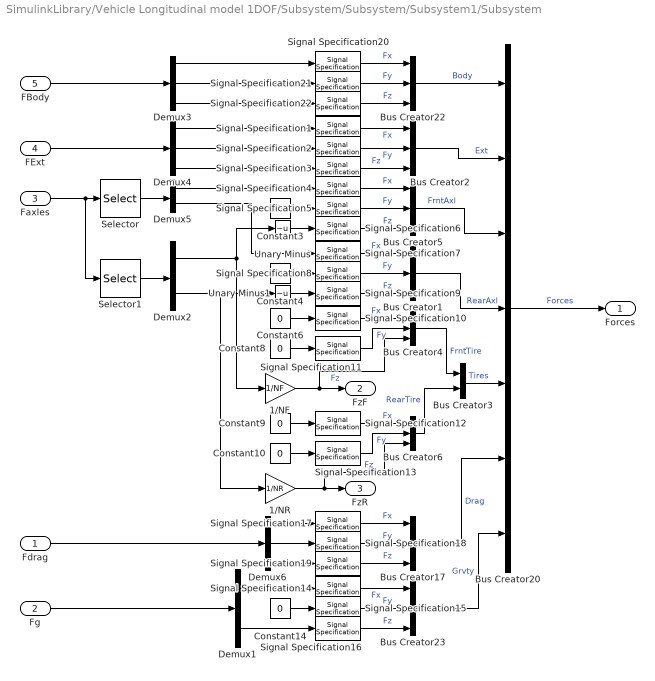
== system SimulinkLibrary/Vehicle Longitudinal model 1DOF/Subsystem/Subsystem/Subsystem1/Subsystem ==
  Fdrag : Inport
  Fg : Inport  Port=2
  Faxles : Inport  Port=3
  FExt : Inport  Port=4
  FBody : Inport  Port=5
  1/NF : Gain  Gain=1/NF
  1/NR : Gain  Gain=1/NR
  Bus Creator{1..2,4..6,17,22..23} (8 alike) : BusCreator  Inputs=3
  Bus Creator20 : BusCreator  Inputs=7
  Bus Creator3 : BusCreator  Inputs=2
  Constant{3..4,6,8..10,14} (7 alike) : Constant  Value=0
  Demux1 : Demux  Outputs=2
  Demux2 : Demux  Outputs=2
  Demux3 : Demux  Outputs=3
  Demux4 : Demux  Outputs=3
  Demux5 : Demux  Outputs=2
  Demux6 : Demux  Outputs=3
  Selector : Selector  NumberOfDimensions=2  InputPortWidth=3  IndexOptions=Select all,Index vector (dialog)  Indices=[1],1  OutputSizes=1,1
  Selector1 : Selector  NumberOfDimensions=2  InputPortWidth=3  IndexOptions=Select all,Index vector (dialog)  Indices=[2],2  OutputSizes=1,1
  Signal Specification{1..22} (22 alike) : SignalSpecification  Unit=N
  Unary Minus : UnaryMinus
  Unary Minus1 : UnaryMinus
  Forces : Outport  VectorParamsAs1DForOutWhenUnconnected=off
  FzF : Outport  Port=2  VectorParamsAs1DForOutWhenUnconnected=off
  FzR : Outport  Port=3  VectorParamsAs1DForOutWhenUnconnected=off
  wires:
  Constant6/1 -> Signal Specification10/1
  Demux4/2 -> Signal Specification2/1
  Signal Specification7/1 -> Bus Creator1/1  "Fx"
  Signal Specification6/1 -> Bus Creator5/3  "Fz"
  Constant3/1 -> Signal Specification5/1
  Constant4/1 -> Signal Specification8/1
  Demux4/1 -> Signal Specification1/1
  Unary Minus1/1 -> Signal Specification9/1
  Constant8/1 -> Signal Specification11/1
  Constant10/1 -> Signal Specification13/1
  1/NR/1 -> FzR/1, Bus Creator6/3  "Fz"
  Selector/1 -> Demux5/1
  Signal Specification12/1 -> Bus Creator6/1  "Fx"
  Demux5/1 -> Signal Specification4/1
  Demux3/1 -> Signal Specification20/1
  Bus Creator3/1 -> Bus Creator20/5  "Tires"
  Fdrag/1 -> Demux6/1
  Faxles/1 -> Selector/1, Selector1/1
  Bus Creator1/1 -> Bus Creator20/4  "RearAxl"
  Bus Creator22/1 -> Bus Creator20/1  "Body"
  Signal Specification11/1 -> Bus Creator4/2  "Fy"
  Signal Specification20/1 -> Bus Creator22/1  "Fx"
  Signal Specification4/1 -> Bus Creator5/1  "Fx"
  Demux6/2 -> Signal Specification18/1
  Constant9/1 -> Signal Specification12/1
  Signal Specification5/1 -> Bus Creator5/2  "Fy"
  Signal Specification1/1 -> Bus Creator2/1  "Fx"
  Bus Creator5/1 -> Bus Creator20/3  "FrntAxl"
  Bus Creator23/1 -> Bus Creator20/7  "Grvty"
  Selector1/1 -> Demux2/1
  Signal Specification2/1 -> Bus Creator2/2  "Fy"
  Demux6/1 -> Signal Specification17/1
  Signal Specification22/1 -> Bus Creator22/3  "Fz"
  Signal Specification15/1 -> Bus Creator23/2  "Fy"
  Signal Specification3/1 -> Bus Creator2/3  "Fz"
  Signal Specification13/1 -> Bus Creator6/2  "Fy"
  Demux6/3 -> Signal Specification19/1
  Demux2/1 -> Unary Minus/1, 1/NF/1
  1/NF/1 -> FzF/1, Bus Creator4/3  "Fz"
  Signal Specification9/1 -> Bus Creator1/3  "Fz"
  Signal Specification14/1 -> Bus Creator23/1  "Fx"
  FBody/1 -> Demux3/1
  Bus Creator20/1 -> Forces/1  "Forces"
  Demux1/1 -> Signal Specification14/1
  Signal Specification18/1 -> Bus Creator17/2  "Fy"
  Bus Creator2/1 -> Bus Creator20/2  "Ext"
  Demux4/3 -> Signal Specification3/1
  Unary Minus/1 -> Signal Specification6/1
  Demux5/2 -> Signal Specification7/1
  Bus Creator4/1 -> Bus Creator3/1  "FrntTire"
  Signal Specification10/1 -> Bus Creator4/1  "Fx"
  Demux3/2 -> Signal Specification21/1
  Constant14/1 -> Signal Specification15/1
  Signal Specification17/1 -> Bus Creator17/1  "Fx"
  Signal Specification21/1 -> Bus Creator22/2  "Fy"
  Bus Creator17/1 -> Bus Creator20/6  "Drag"
  Demux2/2 -> Unary Minus1/1, 1/NR/1
  Bus Creator6/1 -> Bus Creator3/2  "RearTire"
  Signal Specification19/1 -> Bus Creator17/3  "Fz"
  Demux1/2 -> Signal Specification16/1
  Signal Specification8/1 -> Bus Creator1/2  "Fy"
  Signal Specification16/1 -> Bus Creator23/3  "Fz"
  Fg/1 -> Demux1/1
  FExt/1 -> Demux4/1
  Demux3/3 -> Signal Specification22/1

== system SimulinkLibrary/Vehicle Longitudinal model 1DOF/Subsystem/Subsystem/Subsystem3/Subsystem ==
  U,w : Inport
  Theta : Inport  Port=2
  Constant : Constant  Value=0
  Mux3 : Mux  Inputs=3
  Mux4 : Mux  Inputs=3
  Product : Product  Multiplication=Matrix(*)  SaturateOnIntegerOverflow=on  OutDataTypeStr=Inherit: Same as first input
  Rotation Angles to Direction Cosine Matrix : sharedtransform/Rotation Angles to Direction Cosine Matrix  rotationOrder=ZYX  aMode=aMode
      settings: SourceProductBaseCode=AE,PW,DR,MT,UV,VE
  Selector : Selector  InputPortWidth=2  IndexOptions=Index vector (dialog)  Indices=1  OutputSizes=1
  Selector1 : Selector  InputPortWidth=3  IndexOptions=Index vector (dialog)  Indices=[1 3]  OutputSizes=1
  Selector2 : Selector  InputPortWidth=2  IndexOptions=Index vector (dialog)  Indices=2  OutputSizes=1
  Transpose : Math  Operator=transpose  SignedPower=on  SaturateOnIntegerOverflow=on
  Ue,we : Outport  Unit=m/s  VectorParamsAs1DForOutWhenUnconnected=off
  wires:
  Mux4/1 -> Product/2
  Mux3/1 -> Rotation Angles to Direction Cosine Matrix/1
  Transpose/1 -> Product/1
  Theta/1 -> Mux3/2
  U,w/1 -> Selector2/1, Selector/1
  Selector2/1 -> Mux4/3
  Rotation Angles to Direction Cosine Matrix/1 -> Transpose/1
  Selector1/1 -> Ue,we/1
  Product/1 -> Selector1/1
  Selector/1 -> Mux4/1
  Constant/1 -> Mux3/3, Mux4/2, Mux3/1

== system SimulinkLibrary/Vehicle Longitudinal model 1DOF/Subsystem/Subsystem/Subsystem4/Subsystem ==
  InertCg : Inport
  BodyCg : Inport  Port=2
  Forces : Inport  Port=3
  Moments : Inport  Port=4
  Bus Creator1 : BusCreator  Inputs=2
  Bus Creator2 : BusCreator  Inputs=2
  Bus Creator3 : BusCreator  Inputs=3
  Bus Creator4 : BusCreator  Inputs=1
  Bus Creator5 : BusCreator  Inputs=2
  Bus Selector : BusSelector  OutputSignals=Cg.Vel.Zdot
  Bus Selector1 : BusSelector  OutputSignals=Cg.Vel.xdot,Cg.Acc.ax
  Bus Selector2 : BusSelector  OutputSignals=Ext.Fx,Drag.Fx,FrntAxl.Fx,RearAxl.Fx
  Constant : Constant  Value=m*g
  Constant1 : Constant  Value=m
  Demux : Demux
  Mux : Mux
  Product : Product
  Product1 : Product  Inputs=3
  Product8 : Product
  Signal Specification{1..3,5..9} (8 alike) : SignalSpecification  Unit=W
  Signal Specification4 : SignalSpecification  Unit=m/s^2
  Subsystem : Subsystem
  Terminator : Terminator
  Unary Minus : UnaryMinus
  Unary Minus1 : UnaryMinus
  Unit Conversion : UnitConversion
  Pwr : Outport  VectorParamsAs1DForOutWhenUnconnected=off
  wires:
  Signal Specification1/1 -> Bus Creator3/1  "PwrFxExt"
  Bus Selector2/2 -> Mux/2  "<Fx>"
  InertCg/1 -> Bus Selector/1
  Signal Specification3/1 -> Bus Creator1/1  "PwrExt"
  Bus Creator2/1 -> Pwr/1  "Pwr"
  Bus Selector2/4 -> Mux/4  "<Fx>"
  Product8/1 -> Demux/1
  Forces/1 -> Bus Selector2/1
  Moments/1 -> Terminator/1
  Demux/3 -> Signal Specification8/1
  Bus Creator5/1 -> Subsystem/3(PwrStored)
  Unary Minus/1 -> Signal Specification7/1
  Bus Selector1/2 -> Unit Conversion/1  "<ax>"
  Product1/1 -> Signal Specification5/1
  BodyCg/1 -> Bus Selector1/1
  Signal Specification4/1 -> Product1/3
  Unary Minus1/1 -> Signal Specification6/1
  Mux/1 -> Product8/1
  Constant1/1 -> Product1/1
  Bus Selector2/3 -> Mux/3  "<Fx>"
  Bus Creator1/1 -> Bus Creator2/1  "Pwr"
  Product/1 -> Unary Minus1/1
  Bus Creator4/1 -> Subsystem/2(PwrNotTrnsfrd)
  Unit Conversion/1 -> Signal Specification4/1
  Bus Selector2/1 -> Mux/1  "<Fx>"
  Demux/2 -> Unary Minus/1, Signal Specification2/1
  Bus Creator3/1 -> Subsystem/1(PwrTrnsfrd)
  Bus Selector1/1 -> Product8/2, Product1/2  "<xdot>"
  Constant/1 -> Product/1
  Signal Specification7/1 -> Bus Creator4/1  "PwrFxDrag"
  Subsystem/1(PwrInfo) -> Bus Creator2/2  "PwrInfo"
  Demux/1 -> Signal Specification3/1, Signal Specification1/1
  Signal Specification6/1 -> Bus Creator5/1  "PwrStoredGrvty"
  Signal Specification5/1 -> Bus Creator5/2  "PwrStoredxdot"
  Bus Selector/1 -> Product/2  "<Zdot>"
  Demux/4 -> Signal Specification9/1
  Signal Specification9/1 -> Bus Creator3/3  "PwrFwRx"
  Signal Specification8/1 -> Bus Creator3/2  "PwrFwFx"
  Signal Specification2/1 -> Bus Creator1/2  "Drag"

== system SimulinkLibrary/Vehicle Longitudinal model 1DOF/Subsystem/Subsystem/Subsystem5/Subsystem ==
  InertCg : Inport
  BdyFrmCg : Inport  Port=2
  Forces : Inport  Port=3
  Power : Inport  Port=4
  Moments : Inport  Port=5
  WhlAngF : Inport  Port=6
  WhlAngR : Inport  Port=7
  Bus Creator1 : BusCreator  Inputs=6
  Bus Creator2 : BusCreator  Inputs=3
  Bus Creator3 : BusCreator  Inputs=2
  Bus Creator4 : BusCreator  Inputs=2
  Bus Selector : BusSelector  OutputSignals=Pwr,PwrInfo
  Demux : Demux  Outputs=2
  Demux1 : Demux  Outputs=2
  Subsystem : Subsystem  mask{R_T1=a, R_T2=0, R_T3=h}
      mask prompts: R_T1 "x position from CG to suspension hardpoint:"; R_T2 "y position from CG to suspension hardpoint:"; R_T3 "z position from CG to suspension hardpoint:"
  Subsystem1 : $bdroot/Vehicle Longitudinal model 1DOF/Subsystem/Subsystem/Subsystem5/Subsystem/Subsystem  R_T1=-b  R_T2=0  R_T3=h
  InertFrm : Outport  VectorParamsAs1DForOutWhenUnconnected=off
  BdyFrm : Outport  Port=2  VectorParamsAs1DForOutWhenUnconnected=off
  PwrInfo : Outport  Port=3  VectorParamsAs1DForOutWhenUnconnected=off
  wires:
  Demux1/1 -> Bus Creator4/1  "WhlAngRL"
  Power/1 -> Bus Selector/1  "Pwr"
  Demux/2 -> Bus Creator3/2  "WhlAngFR"
  Bus Creator4/1 -> Subsystem1/3  "Steer"
  Bus Selector/1 -> Bus Creator1/6  "<Pwr>"
  Demux1/2 -> Bus Creator4/2  "WhlAngRR"
  Demux/1 -> Bus Creator3/1  "WhlAngFL"
  WhlAngR/1 -> Demux1/1  "WhlAngR"
  Bus Selector/2 -> PwrInfo/1  "<PwrInfo>"
  WhlAngF/1 -> Demux/1  "WhlAngF"
  InertCg/1 -> Subsystem1/1, Subsystem/1(InertFrmCg), Bus Creator2/1  "Cg"
  Moments/1 -> Bus Creator1/3  "Moments"
  Forces/1 -> Bus Creator1/2  "Forces"
  Subsystem1/1 -> Bus Creator2/3  "RearAxl"
  Subsystem/1(Inertial) -> Bus Creator2/2  "FrntAxl"
  Bus Creator1/1 -> BdyFrm/1  "BdyFrm"
  Bus Creator2/1 -> InertFrm/1  "InertFrm"
  Bus Creator3/1 -> Subsystem/3(Steer)  "Steer"
  BdyFrmCg/1 -> Bus Creator1/1, Subsystem1/2, Subsystem/2(BdyFrmCg)  "Cg"
  Subsystem/2(Body) -> Bus Creator1/4  "FrntAxl"
  Subsystem1/2 -> Bus Creator1/5  "RearAxl"

== system SimulinkLibrary/Vehicle Longitudinal model 1DOF/Subsystem/Subsystem/Subsystem4/Subsystem/Subsystem ==
  PwrTrnsfrd : Inport
  PwrNotTrnsfrd : Inport  Port=2
  PwrStored : Inport  Port=3
  Bus Creator : BusCreator  Inputs=3
  Signal Specification : SignalSpecification  Unit=W
  PwrInfo : Outport  VectorParamsAs1DForOutWhenUnconnected=off
  wires:
  PwrNotTrnsfrd/1 -> Bus Creator/2  "PwrNotTrnsfrd"
  PwrStored/1 -> Bus Creator/3  "PwrStored"
  PwrTrnsfrd/1 -> Bus Creator/1  "PwrTrnsfrd"
  Bus Creator/1 -> Signal Specification/1
  Signal Specification/1 -> PwrInfo/1  "PwrInfo"

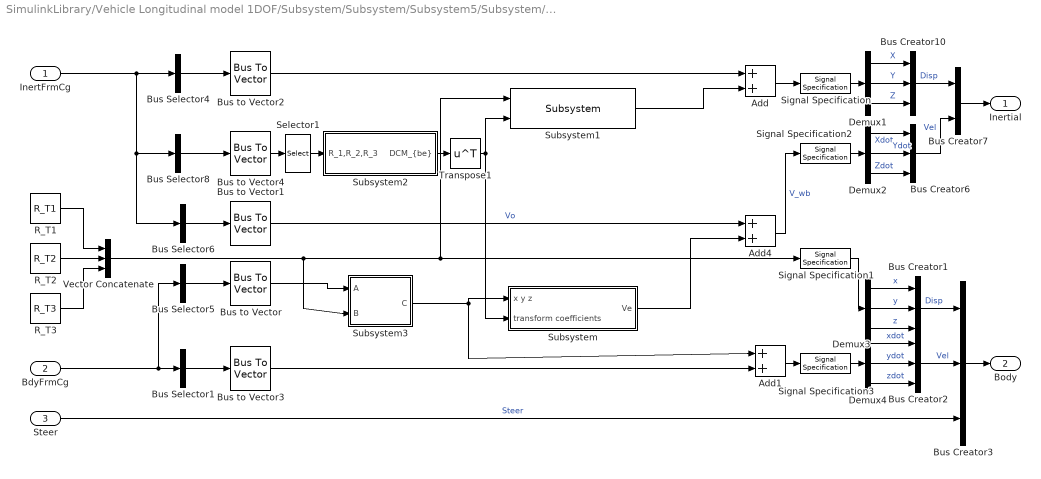
== system SimulinkLibrary/Vehicle Longitudinal model 1DOF/Subsystem/Subsystem/Subsystem5/Subsystem/Subsystem ==
  InertFrmCg : Inport
  BdyFrmCg : Inport  Port=2
  Steer : Inport  Port=3
  Add : Sum
  Add1 : Sum
  Add4 : Sum
  Bus Creator{1..3,6,10} (5 alike) : BusCreator  Inputs=3
  Bus Creator7 : BusCreator  Inputs=2
  Bus Selector1 : BusSelector  OutputSignals=Vel.xdot,Vel.ydot,Vel.zdot  OutputAsBus=on
  Bus Selector4 : BusSelector  OutputSignals=Disp.X,Disp.Y,Disp.Z  OutputAsBus=on
  Bus Selector5 : BusSelector  OutputSignals=AngVel.p,AngVel.q,AngVel.r  OutputAsBus=on
  Bus Selector6 : BusSelector  OutputSignals=Vel.Xdot,Vel.Ydot,Vel.Zdot  OutputAsBus=on
  Bus Selector8 : BusSelector  OutputSignals=Ang.phi,Ang.theta,Ang.psi  OutputAsBus=on
  Bus to Vector{,1..4} (5 alike) : BusToVector
  Demux{1..4} (4 alike) : Demux  Outputs=3
  R_T1 : Constant  Value=R_T1
  R_T2 : Constant  Value=R_T2
  R_T3 : Constant  Value=R_T3
  Selector1 : Selector  InputPortWidth=3  IndexOptions=Index vector (dialog)  Indices=[3 2 1]  OutputSizes=1
  Signal Specification : SignalSpecification  Unit=m
  Signal Specification1 : SignalSpecification  Unit=m
  Signal Specification2 : SignalSpecification  Unit=m/s
  Signal Specification3 : SignalSpecification  Unit=m/s
  Subsystem : Subsystem
  Subsystem1 : $bdroot/Vehicle Longitudinal model 1DOF/Subsystem/Subsystem/Subsystem5/Subsystem/Subsystem/Subsystem  SystemSampleTime=-1  VariantActivationTime=update diagram  Latency=0  AutoFrameSizeCalculation=off
  Subsystem2 : Subsystem
  Subsystem3 : Subsystem
  Transpose1 : Math  Operator=transpose  SignedPower=on  SaturateOnIntegerOverflow=on
  Vector Concatenate : Concatenate  NumInputs=3
  Inertial : Outport  VectorParamsAs1DForOutWhenUnconnected=off
  Body : Outport  Port=2  VectorParamsAs1DForOutWhenUnconnected=off
  wires:
  Demux1/1 -> Bus Creator10/1  "X"
  Bus Selector8/1 -> Bus to Vector4/1
  Subsystem2/1("DCM_{be}") -> Transpose1/1
  Steer/1 -> Bus Creator3/3  "Steer"
  R_T3/1 -> Vector Concatenate/3
  Subsystem1/1 -> Add/2
  Demux2/3 -> Bus Creator6/3  "Zdot"
  Signal Specification3/1 -> Demux4/1
  Add/1 -> Signal Specification/1
  Demux3/2 -> Bus Creator1/2  "y"
  Selector1/1 -> Subsystem2/1(R_1,R_2,R_3)
  Signal Specification1/1 -> Demux3/1
  InertFrmCg/1 -> Bus Selector8/1, Bus Selector6/1, Bus Selector4/1
  Bus to Vector1/1 -> Add4/1  "Vo"
  Bus Selector5/1 -> Bus to Vector/1
  Bus to Vector/1 -> Subsystem3/1(A)
  Bus to Vector2/1 -> Add/1
  Add4/1 -> Signal Specification2/1  "V_wb"
  Bus Selector6/1 -> Bus to Vector1/1
  BdyFrmCg/1 -> Bus Selector1/1, Bus Selector5/1
  Bus to Vector3/1 -> Add1/2
  Subsystem3/1(C) -> Add1/1, Subsystem/1(x y z)
  Bus Creator7/1 -> Inertial/1
  Bus Selector4/1 -> Bus to Vector2/1
  Demux3/1 -> Bus Creator1/1  "x"
  Bus Creator1/1 -> Bus Creator3/1  "Disp"
  Bus Creator2/1 -> Bus Creator3/2  "Vel"
  Demux4/2 -> Bus Creator2/2  "ydot"
  Demux2/1 -> Bus Creator6/1  "Xdot"
  Demux4/3 -> Bus Creator2/3  "zdot"
  Demux1/2 -> Bus Creator10/2  "Y"
  Demux2/2 -> Bus Creator6/2  "Ydot"
  Signal Specification2/1 -> Demux2/1
  Bus Creator6/1 -> Bus Creator7/2  "Vel"
  Bus Creator10/1 -> Bus Creator7/1  "Disp"
  Bus Creator3/1 -> Body/1
  Signal Specification/1 -> Demux1/1
  Bus Selector1/1 -> Bus to Vector3/1
  Add1/1 -> Signal Specification3/1
  R_T2/1 -> Vector Concatenate/2
  Transpose1/1 -> Subsystem1/2, Subsystem/2(transform coefficients)
  Vector Concatenate/1 -> Subsystem3/2(B), Subsystem1/1, Signal Specification1/1
  Subsystem/1(Ve) -> Add4/2
  Demux4/1 -> Bus Creator2/1  "xdot"
  R_T1/1 -> Vector Concatenate/1
  Demux3/3 -> Bus Creator1/3  "z"
  Bus to Vector4/1 -> Selector1/1
  Demux1/3 -> Bus Creator10/3  "Z"

== system SimulinkLibrary/Vehicle Longitudinal model 1DOF/Subsystem/Subsystem/Subsystem5/Subsystem/Subsystem/Subsystem ==
  x y z : Inport
  transform coefficients : Inport  Port=2
  Product : Product  Multiplication=Matrix(*)  InputSameDT=on  SaturateOnIntegerOverflow=on  OutDataTypeStr=Inherit: Same as first input
  Reshape1 : Reshape  OutputDimensionality=Column vector (2-D)
  Reshape2 : Reshape
  Ve : Outport  VectorParamsAs1DForOutWhenUnconnected=off
  wires:
  Reshape1/1 -> Product/2
  transform coefficients/1 -> Product/1
  x y z/1 -> Reshape1/1
  Product/1 -> Reshape2/1
  Reshape2/1 -> Ve/1

== system SimulinkLibrary/Vehicle Longitudinal model 1DOF/Subsystem/Subsystem/Subsystem5/Subsystem/Subsystem/Subsystem2 ==
  R_1,R_2,R_3 : Inport  Unit=rad  PortDimensions=3
  Fcn11 : Fcn  Expr=u(5)*u(4)
  Fcn12 : Fcn  Expr=u(5)*u(1)
  Fcn13 : Fcn  Expr=-u(2)
  Fcn21 : Fcn  Expr=u(3)*u(2)*u(4) - u(6)*u(1)
  Fcn22 : Fcn  Expr=u(3)*u(2)*u(1) + u(6)*u(4)
  Fcn23 : Fcn  Expr=u(3)*u(5)
  Fcn31 : Fcn  Expr=u(6)*u(2)*u(4) + u(3)*u(1)
  Fcn32 : Fcn  Expr=u(6)*u(2)*u(1) - u(3)*u(4)
  Fcn33 : Fcn  Expr=u(6)*u(5)
  Mux : Mux  Inputs=2
  Subsystem : Subsystem
  sincos : Trigonometry  Operator=sincos
  "DCM_{be}" : Outport  Unit=1  PortDimensions=[3,3]  VectorParamsAs1DForOutWhenUnconnected=off
  wires:
  Fcn22/1 -> Subsystem/5(M22)
  Fcn21/1 -> Subsystem/4(M21)
  Fcn31/1 -> Subsystem/7(M31)
  Mux/1 -> Fcn11/1, Fcn12/1, Fcn13/1, Fcn21/1, Fcn32/1, Fcn33/1, Fcn31/1, Fcn23/1, Fcn22/1
  Fcn23/1 -> Subsystem/6(M23)
  Fcn33/1 -> Subsystem/9(M33)
  Fcn32/1 -> Subsystem/8(M32)
  Fcn12/1 -> Subsystem/2(M12)
  Subsystem/1(Matrix) -> "DCM_{be}"/1
  sincos/1 -> Mux/1
  Fcn11/1 -> Subsystem/1(M11)
  Fcn13/1 -> Subsystem/3(M13)
  sincos/2 -> Mux/2
  R_1,R_2,R_3/1 -> sincos/1

== system SimulinkLibrary/Vehicle Longitudinal model 1DOF/Subsystem/Subsystem/Subsystem5/Subsystem/Subsystem/Subsystem3 ==
  A : Inport
  B : Inport  Port=2
  "A " : InportShadow
  "B " : InportShadow  Port=2
  Subsystem1 : $bdroot/Vehicle Longitudinal model 1DOF/Subsystem/Subsystem/Subsystem5/Subsystem/Subsystem/Subsystem3/Subsystem2  SystemSampleTime=-1  VariantActivationTime=update diagram  Latency=0  AutoFrameSizeCalculation=off
  Subsystem2 : Subsystem
  Sum : Sum  Inputs=+|-  InputSameDT=on  SaturateOnIntegerOverflow=on  OutDataTypeStr=Inherit: Same as first input
  C : Outport  VectorParamsAs1DForOutWhenUnconnected=off
  wires:
  B/1 -> Subsystem2/2(B)
  Sum/1 -> C/1
  Subsystem1/1 -> Sum/2
  A/1 -> Subsystem2/1(A)
  "A "/1 -> Subsystem1/1
  "B "/1 -> Subsystem1/2
  Subsystem2/1(Out1) -> Sum/1

== system SimulinkLibrary/Vehicle Longitudinal model 1DOF/Subsystem/Subsystem/Subsystem5/Subsystem/Subsystem/Subsystem2/Subsystem ==
  M11 : Inport  PortDimensions=1
  M12 : Inport  Port=2  PortDimensions=1
  M13 : Inport  Port=3  PortDimensions=1
  M21 : Inport  Port=4  PortDimensions=1
  M22 : Inport  Port=5  PortDimensions=1
  M23 : Inport  Port=6  PortDimensions=1
  M31 : Inport  Port=7  PortDimensions=1
  M32 : Inport  Port=8  PortDimensions=1
  M33 : Inport  Port=9  PortDimensions=1
  Reshape (9) to [3x3] column-major : Reshape  OutputDimensionality=Customize  OutputDimensions=[3,3]
  Vector Concatenate : Concatenate  NumInputs=9
  Matrix : Outport  PortDimensions=[3 3]  VectorParamsAs1DForOutWhenUnconnected=off
  wires:
  M11/1 -> Vector Concatenate/1
  M12/1 -> Vector Concatenate/4
  M32/1 -> Vector Concatenate/6
  M13/1 -> Vector Concatenate/7
  Reshape (9) to [3x3] column-major/1 -> Matrix/1
  Vector Concatenate/1 -> Reshape (9) to [3x3] column-major/1
  M22/1 -> Vector Concatenate/5
  M23/1 -> Vector Concatenate/8
  M31/1 -> Vector Concatenate/3
  M21/1 -> Vector Concatenate/2
  M33/1 -> Vector Concatenate/9

== system SimulinkLibrary/Vehicle Longitudinal model 1DOF/Subsystem/Subsystem/Subsystem5/Subsystem/Subsystem/Subsystem3/Subsystem2 ==
  A : Inport
  B : Inport  Port=2
  Demux : Demux  Outputs=3
  Demux1 : Demux  Outputs=3
  Mux : Mux  Inputs=3
  i x j : Product  InputSameDT=on  SaturateOnIntegerOverflow=on  OutDataTypeStr=Inherit: Same as first input
  j x k : Product  InputSameDT=on  SaturateOnIntegerOverflow=on  OutDataTypeStr=Inherit: Same as first input
  k x i : Product  InputSameDT=on  SaturateOnIntegerOverflow=on  OutDataTypeStr=Inherit: Same as first input
  Out1 : Outport  VectorParamsAs1DForOutWhenUnconnected=off
  wires:
  B/1 -> Demux1/1
  i x j/1 -> Mux/3
  Demux/2 -> j x k/1
  Mux/1 -> Out1/1
  Demux1/1 -> k x i/2
  j x k/1 -> Mux/1
  Demux/1 -> i x j/1
  Demux/3 -> k x i/1
  Demux1/2 -> i x j/2
  A/1 -> Demux/1
  k x i/1 -> Mux/2
  Demux1/3 -> j x k/2

== stateflow chart SimulinkLibrary/Blend/Chart ==
  state Sig1Active
    entry:
    SigOut = SigIn1;
  state Sig2Active
    entry:
    SigOut = SigIn2;
  state INCREMENT
    entry:
    SigOut = SigOut + IncRate;
  state DECREMENT
    entry:
    SigOut = SigOut + DecRate;
  state INCREMENT1
    entry:
    SigOut = SigOut + IncRate;
  state DECREMENT1
    entry:
    SigOut = SigOut + DecRate;
  (default) -> (junction 75)
  (junction 75) -> (junction 77) [order 2]
  (junction 75) -> Sig1Active [order 1] : [Swt ==0] %Sig1 selected
  (junction 77) -> Sig2Active
  (junction 64) -> Sig1Active
  (junction 44) -> Sig2Active
  (junction 62) -> (junction 64)
  (junction 37) -> (junction 44)
  Sig2Active -> (junction 72)
  (junction 72) -> Sig2Active [order 2]
  Sig1Active -> (junction 69)
  (junction 69) -> Sig1Active [order 2]
  (junction 69) -> (junction 18) [order 1] : [Swt ==1] % Switch to sig2
  (junction 72) -> (junction 51) [order 1] : [Swt ==0] % Switch to sig1
  (junction 18) -> (junction 21) [order 1] : [SigIn2 > SigIn1]
  (junction 18) -> DECREMENT [order 2]
  (junction 21) -> INCREMENT
  (junction 51) -> (junction 53) [order 1] : [SigIn1 > SigIn2]
  (junction 51) -> DECREMENT1 [order 2]
  (junction 53) -> INCREMENT1
  DECREMENT -> DECREMENT [order 2]
  INCREMENT -> INCREMENT [order 2]
  DECREMENT -> (junction 34) [order 1] : [SigOut <= SigIn2 ]
  INCREMENT -> (junction 40) [order 1] : [SigOut >= SigIn2 ]
  DECREMENT1 -> DECREMENT1 [order 2]
  INCREMENT1 -> INCREMENT1 [order 2]
  (junction 34) -> (junction 40)
  (junction 40) -> (junction 37)
  DECREMENT1 -> (junction 60) [order 1] : [SigOut <= SigIn1 ]
  INCREMENT1 -> (junction 59) [order 1] : [SigOut >= SigIn1 ]
  (junction 60) -> (junction 62)
  (junction 59) -> (junction 60)
  data: Swt input; SigOut output; SigIn1 input; SigIn2 input; IncRate input; DecRate input
